simulink model "Ejercicio_6"  (Simulink 9.2)
settings: Solver=ode4  StartTime=0.0  StopTime=30.0  FixedStep=0.05  RelTol=1e-3
settings Model: Creator=hathaway  LastModifiedBy=hathaway
settings DataIOCC: LimitDataPoints=off  SaveFormat=Dataset  SignalLoggingSaveFormat=Dataset
settings OptimizationCC: LifeSpan=auto
settings DebuggingCC: UnderspecifiedInitializationDetection=Simplified  MergeDetectMultiDrivingBlocksExec=error  FcnCallInpInsideContextMsg=error  StateNameClashWarn=none  SFUnexpectedBacktrackingDiag=error  SFNoUnconditionalDefaultTransitionDiag=error  SFExecutionAtInitializationDiag=warning
settings HardwareCC: ProdBitPerPointer=64  ProdBitPerSizeT=64  ProdBitPerPtrDiffT=64  ProdLargestAtomicFloat=Float  ProdIntDivRoundTo=Zero  ProdEndianess=LittleEndian  ProdWordSize=64  ProdHWDeviceType=Intel->x86-64 (Windows64)
settings ModelReferenceCC: PropagateSignalLabelsOutOfModel=on
settings SFSimCC: SimUseLocalCustomCode=on
settings RTWCC: RTWUseLocalCustomCode=on
settings CodeAppCC: StateflowObjectComments=off
settings GRTTargetCC: TargetLangStandard=C99 (ISO)  GeneratePreprocessorConditionals=Use local settings  CombineOutputUpdateFcns=on  GRTInterface=off
settings ConfigComp: CovMetricSettings=dwe  CovHtmlReporting=off  CovSaveCumulativeToWorkspaceVar=off  CovSaveSingleToWorkspaceVar=off  CovExternalEMLEnable=on

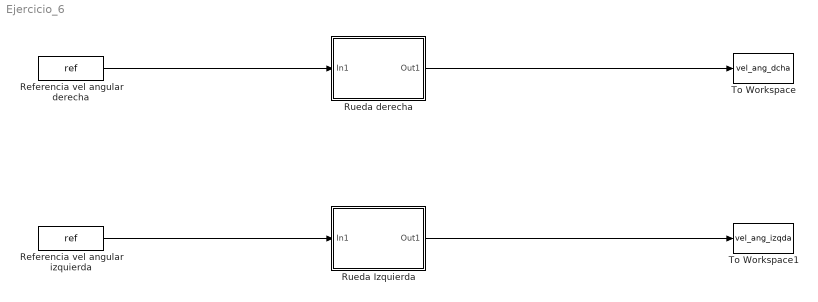
== system Ejercicio_6 ==
  Referencia vel angular derecha : FromWorkspace  VariableName=ref  SampleTime=0
  Referencia vel angular izquierda : FromWorkspace  VariableName=ref  SampleTime=0
  Rueda Izquierda : Subsystem  mask{k=0.2, tau=0.09, kp=3}
      mask prompts: k "Valor ganancia del motor:"; tau "Valor cte tiempo motor:"; kp "Valor ganancia regulador P:"
  Rueda derecha : Subsystem  mask{k=0.2, tau=0.09, kp=3}
      mask prompts: k "Valor ganancia del motor:"; tau "Valor cte tiempo motor:"; kp "Valor ganancia regulador P:"
  To Workspace : ToWorkspace  VariableName=vel_ang_dcha  SaveFormat=Timeseries  SampleTime=-1
  To Workspace1 : ToWorkspace  VariableName=vel_ang_izqda  SaveFormat=Timeseries  SampleTime=-1
  wires:
  Referencia vel angular derecha/1 -> Rueda derecha/1(In1)
  Rueda derecha/1(Out1) -> To Workspace/1
  Rueda Izquierda/1(Out1) -> To Workspace1/1
  Referencia vel angular izquierda/1 -> Rueda Izquierda/1(In1)

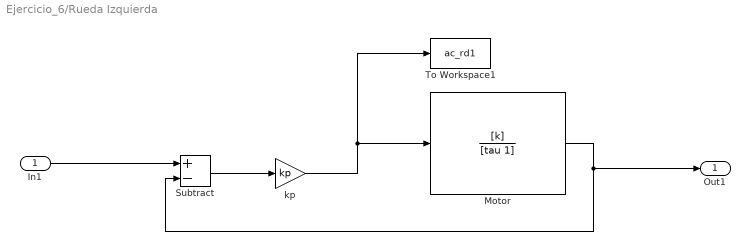
== system Ejercicio_6/Rueda Izquierda ==
  In1 : Inport
  Motor : TransferFcn  Numerator=[k]  Denominator=[tau 1]
  Subtract : Sum  Inputs=+-
  To Workspace1 : ToWorkspace  VariableName=ac_rd1  SaveFormat=Timeseries  SampleTime=-1
  kp : Gain  Gain=kp
  Out1 : Outport
  wires:
  In1/1 -> Subtract/1
  Subtract/1 -> kp/1
  kp/1 -> Motor/1, To Workspace1/1
  Motor/1 -> Subtract/2, Out1/1

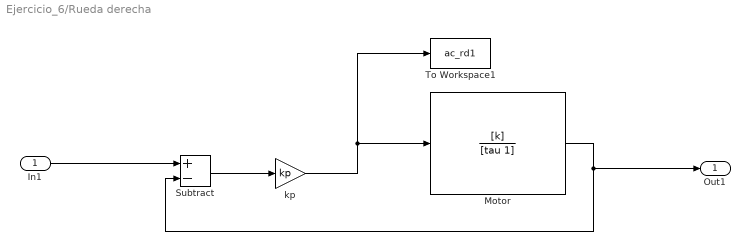
== system Ejercicio_6/Rueda derecha ==
  In1 : Inport
  Motor : TransferFcn  Numerator=[k]  Denominator=[tau 1]
  Subtract : Sum  Inputs=+-
  To Workspace1 : ToWorkspace  VariableName=ac_rd1  SaveFormat=Timeseries  SampleTime=-1
  kp : Gain  Gain=kp
  Out1 : Outport
  wires:
  Motor/1 -> Out1/1, Subtract/2
  kp/1 -> To Workspace1/1, Motor/1
  Subtract/1 -> kp/1
  In1/1 -> Subtract/1
